simulink model "ADAS_Main_ClosedLoop"  (R2026a)
settings: Solver=FixedStepDiscrete  StopTime=20
InitFcn:
  | createLidarActorProfiles;
  | % L3/L4 closed-loop ego initial condition, READ FROM THE TEST-1 FIXTURE
  | % (not hard-coded in the vehicle model, which stays reusable)
  | clS = load('D:\AutonomousDriving\D_scenarios\V2_0_ClosedLoop_Test9_TwoObstacles_WideRoad.mat');
  | clA = clS.data.ActorSpecifications([clS.data.ActorSpecifications.ActorID] == clS.data.EgoCarId);
  | CL_EGO_IC = [clA.Position(1); clA.Position(2); clA.Yaw*pi/180; clA.Speed(1)];
  | clear clS clA
  | % Non-virtual ego-pose bus type. A MATLAB Function block (Extract_Ego_Kinematics)
  | % cannot accept a VIRTUAL bus, so the Bus Creator must emit a defined Simulink.Bus.
  | % Shape copied from the installed validator contract and from BusActorsActors.
  | clN = {'ActorID','Position','Velocity','Roll','Pitch','Yaw','AngularVelocity'};
  | clD = {[1 1],[1 3],[1 3],[1 1],[1 1],[1 1],[1 3]};
  | clEls = Simulink.BusElement.empty(0,1);
  | for clI = 1:7
  |   clE = Simulink.BusElement; clE.Name = clN{clI}; clE.Dimensions = clD{clI}; clE.DataType = 'double';
  |   clEls(clI,1) = clE;
  | end
  | BusEgoPose_CL = Simulink.Bus; BusEgoPose_CL.Elements = clEls;
  | clear clN clD clEls clE clI
StopFcn:
  | cl_plot_closedloop_trajectory;
model workspace (MAT data in the model file):
  firstWarning = 1
  originalScenarioChecksum = '71EAF3DF157DF5A35F75811B676F8B0F'
undefined symbols (not defined in the file): driving, matlabshared
libraries: drivingscenarioandsensors x3, lidarlib x1
(part 2 of 7)

== matlab function ADAS_Main_ClosedLoop/Sensor_Fusion/Normalize_Detections ==
  data: visionBus input; visionMeas output; radarBus input; lidarDet input; numLidarDet input; numVision output; radarMeas output; numRadar output; lidarMeas output; numLidar output
function [visionMeas, numVision, radarMeas, numRadar, lidarMeas, numLidar] = ...
    Normalize_Detections(visionBus, radarBus, lidarDet, numLidarDet)
%#codegen
% NORMALIZE_DETECTIONS  Stage F2 of Sensor Fusion: normalisation ONLY.
%
% Unpacks the Vision and Radar detection buses and the LiDAR detection matrix
% into three fixed-size measurement tables in the common ego frame.
%
% THIS STAGE DOES NOT: associate, gate, fuse, score, inflate covariance,
% classify, estimate velocity, or discard anything.
%
% NOTHING IS REJECTED. Every emitted detection is preserved. Covariance
% validity is reported per detection via CovValid flags so that the later
% fusion stage decides what to do. "no detection" and "detection with invalid
% covariance" are therefore never confused: the former has Valid = 0, the
% latter has Valid = 1 with PosCovValid = 0.
%
% MEASUREMENT SUBSPACES - only what each sensor actually measures:
%   Vision : x, y, vx, vy  (+ their 2x2 covariances)
%   Radar  : x, y, vx, vy  (+ their 2x2 covariances) + SNR
%   LiDAR  : the validated [256x20] detection row, passed through unchanged
%   Radar z / vz and Vision z / vz are NOT normalised. Radar elevation is off,
%   so its z is a nominal constant, not a measurement; vz is unobserved by both
%   (reported variance 100). Manufacturing them here would invent capability
%   the sensors do not have.
%
% SCENARIO INDEPENDENCE: reads only measurements and measurement covariance.
% It does not reference ActorID, ClassID, MaterialID, Clusters, actor poses,
% actor profiles, TargetIndex, or any scenario property. Loop bounds are the
% declared sensor interface capacities, never an actor count.

MAX_V  = 50;   NCOL_V = 13;   % Vision capacity  = MaxNumDetections
MAX_R  = 50;   NCOL_R = 14;   % Radar  capacity  = MaxNumReports
MAX_L  = 256;  NCOL_L = 21;   % LiDAR  capacity  = LiDARDetections rows

% Vision / Radar table columns
%   1 Valid
%   2 PosX          m
%   3 PosY          m
%   4 PosCovXX      m^2
%   5 PosCovYY      m^2
%   6 PosCovXY      m^2
%   7 VelX          m/s
%   8 VelY          m/s
%   9 VelCovXX      m^2/s^2
%  10 VelCovYY      m^2/s^2
%  11 VelCovXY      m^2/s^2
%  12 PosCovValid   0/1   2x2 position covariance is finite and positive definite
%  13 VelCovValid   0/1   2x2 velocity covariance is finite and positive definite
%  14 SNR           dB    (Radar table only)
%
% LiDAR table columns
%   1..20  the LiDARDetections row, unchanged
%   21     PosCovValid  0/1   from columns 5,6,7

visionMeas = zeros(MAX_V, NCOL_V);
radarMeas  = zeros(MAX_R, NCOL_R);
lidarMeas  = zeros(MAX_L, NCOL_L);

%% ---- Vision -------------------------------------------------------------
nV = double(visionBus.NumDetections);
if nV < 0,     nV = 0;     end
if nV > MAX_V, nV = MAX_V;  end
for i = 1:MAX_V
    if i > nV
        continue
    end
    m = visionBus.Detections(i).Measurement;
    C = visionBus.Detections(i).MeasurementNoise;
    pxx = double(C(1,1)); pyy = double(C(2,2)); pxy = double(C(1,2));
    vxx = double(C(4,4)); vyy = double(C(5,5)); vxy = double(C(4,5));
    visionMeas(i, 1)  = 1;
    visionMeas(i, 2)  = double(m(1));
    visionMeas(i, 3)  = double(m(2));
    visionMeas(i, 4)  = pxx;
    visionMeas(i, 5)  = pyy;
    visionMeas(i, 6)  = pxy;
    visionMeas(i, 7)  = double(m(4));
    visionMeas(i, 8)  = double(m(5));
    visionMeas(i, 9)  = vxx;
    visionMeas(i, 10) = vyy;
    visionMeas(i, 11) = vxy;
    if isPD2(pxx, pyy, pxy), visionMeas(i, 12) = 1; end
    if isPD2(vxx, vyy, vxy), visionMeas(i, 13) = 1; end
end
numVision = uint32(nV);

%% ---- Radar --------------------------------------------------------------
nR = double(radarBus.NumDetections);
if nR < 0,     nR = 0;     end
if nR > MAX_R, nR = MAX_R;  end
for i = 1:MAX_R
    if i > nR
        continue
    end
    m = radarBus.Detections(i).Measurement;
    C = radarBus.Detections(i).MeasurementNoise;
    pxx = double(C(1,1)); pyy = double(C(2,2)); pxy = double(C(1,2));
    vxx = double(C(4,4)); vyy = double(C(5,5)); vxy = double(C(4,5));
    radarMeas(i, 1)  = 1;
    radarMeas(i, 2)  = double(m(1));
    radarMeas(i, 3)  = double(m(2));
    radarMeas(i, 4)  = pxx;
    radarMeas(i, 5)  = pyy;
    radarMeas(i, 6)  = pxy;
    radarMeas(i, 7)  = double(m(4));
    radarMeas(i, 8)  = double(m(5));
    radarMeas(i, 9)  = vxx;
    radarMeas(i, 10) = vyy;
    radarMeas(i, 11) = vxy;
    if isPD2(pxx, pyy, pxy), radarMeas(i, 12) = 1; end
    if isPD2(vxx, vyy, vxy), radarMeas(i, 13) = 1; end
    % SNR only. No other ObjectAttributes field is read.
    radarMeas(i, 14) = double(radarBus.Detections(i).ObjectAttributes.SNR);
end
numRadar = uint32(nR);

%% ---- LiDAR --------------------------------------------------------------
nL = double(numLidarDet);
if nL < 0,     nL = 0;     end
if nL > MAX_L, nL = MAX_L;  end
for i = 1:MAX_L
    if i > nL
        continue
    end
    for c = 1:20
        lidarMeas(i, c) = lidarDet(i, c);
    end
    if isPD2(lidarDet(i,5), lidarDet(i,6), lidarDet(i,7))
        lidarMeas(i, 21) = 1;
    end
end
numLidar = uint32(nL);

end

% ===========================================================================
function tf = isPD2(a, b, c)
% 2x2 symmetric [a c; c b] is positive definite iff a > 0 and det > 0.
tf = false;
if isfinite(a) && isfinite(b) && isfinite(c)
    if a > 0 && b > 0 && (a*b - c*c) > 0
        tf = true;
    end
end
end

== matlab function ADAS_Main_ClosedLoop/Sensor_Fusion/Associate_Detections ==
  data: visionMeas input; groups output; numVision input; radarMeas input; numRadar input; lidarMeas input; numLidar input; numGroups output
function [groups, numGroups] = Associate_Detections( ...
    visionMeas, numVision, radarMeas, numRadar, lidarMeas, numLidar)
%#codegen
% ASSOCIATE_DETECTIONS  Stage F3: gating + compatibility grouping ONLY.
%
% THIS STAGE DOES NOT: fuse positions, fuse velocities, compute a support
% score, fuse class, or discard any detection. It only decides which sensor
% measurements are compatible enough to represent the same physical object.
%
% EVERY detection appears in exactly one group. A detection with no compatible
% partner forms a singleton group - that is the expected outcome for the large
% majority, because Radar and Vision have narrow forward fields of view while
% LiDAR is 360 deg. A high LiDAR count must never be forced into matches.
%
% GATE
%   2-D Mahalanobis on position only:
%       d2 = delta' * inv(R1' + R2') * delta        delta = [dx; dy]
%       compatible iff d2 < GATE_CHI2
%   Position only, because z is unobserved by Vision and nominal-only for
%   Radar, and velocity is unavailable from LiDAR.
%
% LiDAR REFERENCE-POINT TERM  B
%   LiDAR reports the centroid of visible surfaces, not the object centre.
%   Modelling that offset as uniform over the object's line-of-sight depth D
%   gives variance D^2/12 (the second moment of a uniform offset). Applied
%   ALONG the line of sight only, then rotated into ego coordinates.
%
%   Applied ONLY when ExtentUntrusted (LiDARFlags bit 8) is set. When the
%   extents are trustworthy the LiDAR block's own GAMMA_ALONG = 0.25 term is
%   already 87% of 1/(2*sqrt(3)) = 0.2887, i.e. it already implements
%   approximately this same variance using the yaw-projected depth
%   D_los = |L*cos(theta)| + |W*sin(theta)|, so adding B there would
%   double-count.
%
%   When ExtentUntrusted, the PCA extents have collapsed and that projection is
%   meaningless, so D_los = max(Length, Width) is used as a geometric proxy.
%   KNOWN LIMITATION: for a long object viewed end-on this under-estimates the
%   true line-of-sight depth.
%
% GROUPING
%   Mutual-best matching, which is symmetric and therefore order-independent:
%   a pair is joined only if each is the other's lowest-d2 compatible partner.
%   Ties break on the lower index. A group holds at most one detection per
%   sensor. Before a group keeps both a Vision and a Radar member they must
%   also be compatible with each other (clique, never a chain); if not, the
%   weaker link is dropped and ChainSplit is flagged.
%
% SCENARIO INDEPENDENCE: reads only measurements, covariances and LiDAR
% observation flags. No actor identity, class, count or scenario geometry.
% Loop bounds are the declared interface capacities.

MAX_V = 50; MAX_R = 50; MAX_L = 256; MAX_G = 356; NCOL_G = 6;
GATE_CHI2 = 9.21;        % chi-square, 2 DOF, 0.99

% LiDARMeas column map
CL_X = 2; CL_Y = 3; CL_CXX = 5; CL_CYY = 6; CL_CXY = 7;
CL_LEN = 9; CL_WID = 10; CL_FLAGS = 20; CL_COVOK = 21;
FLAG_EXTENT_UNTRUSTED = uint32(8);

groups    = zeros(MAX_G, NCOL_G);
numGroups = uint32(0);

nV = double(numVision); if nV > MAX_V, nV = MAX_V; end; if nV < 0, nV = 0; end
nR = double(numRadar);  if nR > MAX_R, nR = MAX_R; end; if nR < 0, nR = 0; end
nL = double(numLidar);  if nL > MAX_L, nL = MAX_L; end; if nL < 0, nL = 0; end

%% ---- gather positions, covariances and per-detection covariance validity
vx = zeros(MAX_V,1); vy = zeros(MAX_V,1);
vxx = zeros(MAX_V,1); vyy = zeros(MAX_V,1); vxy = zeros(MAX_V,1);
vok = false(MAX_V,1);
for i = 1:nV
    vx(i) = visionMeas(i,2);  vy(i) = visionMeas(i,3);
    vxx(i)= visionMeas(i,4);  vyy(i)= visionMeas(i,5);  vxy(i)= visionMeas(i,6);
    vok(i)= visionMeas(i,12) == 1;
end

rx = zeros(MAX_R,1); ry = zeros(MAX_R,1);
rxx = zeros(MAX_R,1); ryy = zeros(MAX_R,1); rxy = zeros(MAX_R,1);
rok = false(MAX_R,1);
for i = 1:nR
    rx(i) = radarMeas(i,2);  ry(i) = radarMeas(i,3);
    rxx(i)= radarMeas(i,4);  ryy(i)= radarMeas(i,5);  rxy(i)= radarMeas(i,6);
    rok(i)= radarMeas(i,12) == 1;
end

lx = zeros(MAX_L,1); ly = zeros(MAX_L,1);
lxx = zeros(MAX_L,1); lyy = zeros(MAX_L,1); lxy = zeros(MAX_L,1);
lok = false(MAX_L,1); lbias = false(MAX_L,1);
for i = 1:nL
    px = lidarMeas(i,CL_X);  py = lidarMeas(i,CL_Y);
    lx(i) = px;  ly(i) = py;
    cxx = lidarMeas(i,CL_CXX); cyy = lidarMeas(i,CL_CYY); cxy = lidarMeas(i,CL_CXY);
    if bitand(uint32(lidarMeas(i,CL_FLAGS)), FLAG_EXTENT_UNTRUSTED) > 0
        D = lidarMeas(i,CL_LEN);
        if lidarMeas(i,CL_WID) > D, D = lidarMeas(i,CL_WID); end
        bAlong = (D*D)/12;
        az = atan2(py, px);
        ca = cos(az); sa = sin(az);
        cxx = cxx + bAlong*ca*ca;
        cyy = cyy + bAlong*sa*sa;
        cxy = cxy + bAlong*ca*sa;
        lbias(i) = true;
    end
    lxx(i) = cxx; lyy(i) = cyy; lxy(i) = cxy;
    lok(i) = lidarMeas(i,CL_COVOK) == 1;
end

%% ---- pairwise gate
% A detection whose position covariance is not positive definite cannot be
% gated (the Mahalanobis distance is undefined), so it is never associated.
% It is preserved as a singleton and flagged, never discarded.
dVR = zeros(MAX_V, MAX_R); cVR = false(MAX_V, MAX_R);
dVL = zeros(MAX_V, MAX_L); cVL = false(MAX_V, MAX_L);
dRL = zeros(MAX_R, MAX_L); cRL = false(MAX_R, MAX_L);

for i = 1:nV
    for j = 1:nR
        if vok(i) && rok(j)
            [ok, d2] = gate2(vx(i)-rx(j), vy(i)-ry(j), ...
                vxx(i)+rxx(j), vyy(i)+ryy(j), vxy(i)+rxy(j), GATE_CHI2);
            dVR(i,j) = d2; cVR(i,j) = ok;
        end
    end
end
for i = 1:nV
    for j = 1:nL
        if vok(i) && lok(j)
            [ok, d2] = gate2(vx(i)-lx(j), vy(i)-ly(j), ...
                vxx(i)+lxx(j), vyy(i)+lyy(j), vxy(i)+lxy(j), GATE_CHI2);
            dVL(i,j) = d2; cVL(i,j) = ok;
        end
    end
end
for i = 1:nR
    for j = 1:nL
        if rok(i) && lok(j)
            [ok, d2] = gate2(rx(i)-lx(j), ry(i)-ly(j), ...
                rxx(i)+lxx(j), ryy(i)+lyy(j), rxy(i)+lxy(j), GATE_CHI2);
            dRL(i,j) = d2; cRL(i,j) = ok;
        end
    end
end

%% ---- mutual-best matching (symmetric => order-independent)
mVL = zeros(MAX_L,1);   % for each LiDAR, its mutually-best Vision (0 = none)
mRL = zeros(MAX_L,1);   % for each LiDAR, its mutually-best Radar
mVR = zeros(MAX_V,1);   % for each Vision, its mutually-best Radar

for j = 1:nL
    b = bestIn(dVL(:,j), cVL(:,j), nV);
    if b > 0
        bb = bestIn(dVL(b,:)', cVL(b,:)', nL);
        if bb == j, mVL(j) = b; end
    end
end
for j = 1:nL
    b = bestIn(dRL(:,j), cRL(:,j), nR);
    if b > 0
        bb = bestIn(dRL(b,:)', cRL(b,:)', nL);
        if bb == j, mRL(j) = b; end
    end
end
for i = 1:nV
    b = bestIn(dVR(i,:)', cVR(i,:)', nR);
    if b > 0
        bb = bestIn(dVR(:,b), cVR(:,b), nV);
        if bb == i, mVR(i) = b; end
    end
end

%% ---- build groups: LiDAR-anchored first, then leftover Radar/Vision
vUsed = false(MAX_V,1); rUsed = false(MAX_R,1);
g = 0;

for j = 1:nL
    g = g + 1;
    vIdx = mVL(j); rIdx = mRL(j);
    if vIdx > 0 && vUsed(vIdx), vIdx = 0; end
    if rIdx > 0 && rUsed(rIdx), rIdx = 0; end
    fl = 0;
    % clique: a group holding both Vision and Radar needs them compatible too
    if vIdx > 0 && rIdx > 0 && ~cVR(vIdx, rIdx)
        if dVL(vIdx,j) <= dRL(rIdx,j)
            rIdx = 0;
        else
            vIdx = 0;
        end
        fl = fl + 1;                       % ChainSplit
    end
    if ~lok(j), fl = fl + 2; end           % CovInvalid member
    if lbias(j), fl = fl + 4; end          % LiDAR B applied
    if vIdx > 0, vUsed(vIdx) = true; end
    if rIdx > 0, rUsed(rIdx) = true; end
    cnt = 1;
    if vIdx > 0, cnt = cnt + 1; end
    if rIdx > 0, cnt = cnt + 1; end
    groups(g,1) = 1;
    groups(g,2) = vIdx;
    groups(g,3) = rIdx;
    groups(g,4) = j;
    groups(g,5) = cnt;
    groups(g,6) = fl;
end

% Radar not yet grouped: may pair with an ungrouped mutually-best Vision
for i = 1:nR
    if rUsed(i), continue; end
    g = g + 1;
    vIdx = 0;
    for k = 1:nV
        if mVR(k) == i && ~vUsed(k)
            vIdx = k; break
        end
    end
    fl = 0;
    if ~rok(i), fl = fl + 2; end
    if vIdx > 0, vUsed(vIdx) = true; end
    cnt = 1; if vIdx > 0, cnt = 2; end
    groups(g,1) = 1;
    groups(g,2) = vIdx;
    groups(g,3) = i;
    groups(g,4) = 0;
    groups(g,5) = cnt;
    groups(g,6) = fl;
    rUsed(i) = true;
end

% Vision left over: singletons
for i = 1:nV
    if vUsed(i), continue; end
    g = g + 1;
    fl = 0;
    if ~vok(i), fl = fl + 2; end
    groups(g,1) = 1;
    groups(g,2) = i;
    groups(g,3) = 0;
    groups(g,4) = 0;
    groups(g,5) = 1;
    groups(g,6) = fl;
    vUsed(i) = true;
end

numGroups = uint32(g);

end

% ===========================================================================
function [ok, d2] = gate2(dx, dy, sxx, syy, sxy, thr)
ok = false; d2 = 0;
det = sxx*syy - sxy*sxy;
if isfinite(det) && det > 0 && sxx > 0
    d2 = (dx*dx*syy - 2*dx*dy*sxy + dy*dy*sxx)/det;
    if isfinite(d2) && d2 >= 0 && d2 < thr
        ok = true;
    end
end
end

% ===========================================================================
function b = bestIn(d, c, n)
% Lowest d2 among compatible entries 1..n. Ties break on the lower index.
b = 0; bd = 0;
for k = 1:n
    if c(k)
        if b == 0 || d(k) < bd
            b = k; bd = d(k);
        end
    end
end
end

== matlab function ADAS_Main_ClosedLoop/Sensor_Fusion/Fuse_Position ==
  data: visionMeas input; fusedPos output; numVision input; radarMeas input; numRadar input; lidarMeas input; numLidar input; groups input; numGroups input; numFused output
function [fusedPos, numFused] = Fuse_Position( ...
    visionMeas, numVision, radarMeas, numRadar, lidarMeas, numLidar, groups, numGroups)
%#codegen
% FUSE_POSITION  Stage F4: information-form fusion of X/Y position ONLY.
%
% THIS STAGE DOES NOT: fuse velocity, compute a support score, fuse class,
% track, or discard anything. Every group from F3 produces exactly one output
% row, in the same order.
%
% METHOD
%   For a group with two or more usable members, the maximum-likelihood
%   combination of independent simultaneous measurements is the information
%   form:
%       Y = sum_i inv(Ri)          (information matrix)
%       y = sum_i inv(Ri) * zi     (information vector)
%       P = inv(Y),  x = P * y
%   For a singleton the measurement and covariance pass through unchanged.
%   There is no prediction, no process model and no state carried between
%   frames - that belongs to Tracking, not here.
%
% LiDAR REFERENCE-POINT TERM  B
%   Recomputed here with the SAME formula used by Associate_Detections in F3:
%   applied only when ExtentUntrusted (LiDARFlags bit 8), D = max(Length,Width),
%   variance D^2/12 along the line of sight, rotated into ego coordinates.
%   The two stages must stay in sync; the F4 checkpoint verifies this by
%   recomputing B independently and comparing the singleton LiDAR rows.
%
% DEFENSIVE COVARIANCE HANDLING
%   A member whose 2x2 position covariance is not finite and positive definite
%   is NEVER inverted. It is excluded from the information sum and
%   FusionDegraded is flagged. If no member has a usable covariance the
%   detection is still preserved: its raw position is passed through with its
%   own covariance untouched, and the flags say so. Nothing is discarded and
%   no singular matrix is ever used.
%
% SCENARIO INDEPENDENCE: consumes only measurements, covariances, LiDAR
% observation flags and the F3 grouping. No actor identity, class, count or
% scenario geometry. Loop bounds are the declared interface capacities.

MAX_G = 356; NCOL_F = 11;
FLAG_EXTENT_UNTRUSTED = uint32(8);

% LiDARMeas column map
CL_X = 2; CL_Y = 3; CL_CXX = 5; CL_CYY = 6; CL_CXY = 7;
CL_LEN = 9; CL_WID = 10; CL_FLAGS = 20;

% fusedPos columns
%   1 Valid
%   2 PosX          m, ego
%   3 PosY          m, ego
%   4 PosCovXX      m^2
%   5 PosCovYY      m^2
%   6 PosCovXY      m^2
%   7 SensorMask    1 = Vision, 2 = Radar, 4 = LiDAR
%   8 VisionIdx     source row in visionMeas (0 = none)
%   9 RadarIdx      source row in radarMeas  (0 = none)
%  10 LiDARIdx      source row in lidarMeas  (0 = none)
%  11 FusionFlags   1 ChainSplit | 2 CovInvalidMember | 4 LiDARBiasApplied
%                   8 FusionDegraded | 16 OutsideMeasurementBox

fusedPos = zeros(MAX_G, NCOL_F);
numFused = uint32(0);

nG = double(numGroups);
if nG < 0, nG = 0; end
if nG > MAX_G, nG = MAX_G; end

for g = 1:nG
    if groups(g,1) ~= 1
        continue
    end
    vi = groups(g,2);
    ri = groups(g,3);
    li = groups(g,4);
    fl = uint32(groups(g,6));        % inherit ChainSplit / CovInvalid / BiasApplied

    % ---- gather up to three members
    mx = zeros(3,1); my = zeros(3,1);
    ma = zeros(3,1); mb = zeros(3,1); mc = zeros(3,1);
    mUse = false(3,1);
    nMem = 0;
    mask = 0;

    if vi > 0
        nMem = nMem + 1; mask = mask + 1;
        mx(nMem) = visionMeas(vi,2); my(nMem) = visionMeas(vi,3);
        ma(nMem) = visionMeas(vi,4); mb(nMem) = visionMeas(vi,5); mc(nMem) = visionMeas(vi,6);
        mUse(nMem) = isPD2(ma(nMem), mb(nMem), mc(nMem));
    end
    if ri > 0
        nMem = nMem + 1; mask = mask + 2;
        mx(nMem) = radarMeas(ri,2); my(nMem) = radarMeas(ri,3);
        ma(nMem) = radarMeas(ri,4); mb(nMem) = radarMeas(ri,5); mc(nMem) = radarMeas(ri,6);
        mUse(nMem) = isPD2(ma(nMem), mb(nMem), mc(nMem));
    end
    if li > 0
        nMem = nMem + 1; mask = mask + 4;
        px = lidarMeas(li,CL_X); py = lidarMeas(li,CL_Y);
        a = lidarMeas(li,CL_CXX); b = lidarMeas(li,CL_CYY); c = lidarMeas(li,CL_CXY);
        if bitand(uint32(lidarMeas(li,CL_FLAGS)), FLAG_EXTENT_UNTRUSTED) > 0
            D = lidarMeas(li,CL_LEN);
            if lidarMeas(li,CL_WID) > D, D = lidarMeas(li,CL_WID); end
            bAlong = (D*D)/12;
            az = atan2(py, px);
            ca = cos(az); sa = sin(az);
            a = a + bAlong*ca*ca;
            b = b + bAlong*sa*sa;
            c = c + bAlong*ca*sa;
        end
        mx(nMem) = px; my(nMem) = py;
        ma(nMem) = a;  mb(nMem) = b;  mc(nMem) = c;
        mUse(nMem) = isPD2(a, b, c);
    end

    nUse = 0;
    for m = 1:nMem
        if mUse(m), nUse = nUse + 1; end
    end
    if nUse < nMem
        fl = fl + uint32(8);                     % FusionDegraded
    end

    outX = 0; outY = 0; outA = 0; outB = 0; outC = 0;

    if nUse == 0
        % preserve the detection; never invert a singular matrix
        outX = mx(1); outY = my(1);
        outA = ma(1); outB = mb(1); outC = mc(1);
    elseif nUse == 1
        for m = 1:nMem
            if mUse(m)
                outX = mx(m); outY = my(m);
                outA = ma(m); outB = mb(m); outC = mc(m);
            end
        end
    else
        % ---- information form over the usable members
        Yxx = 0; Yyy = 0; Yxy = 0; yx = 0; yy = 0;
        for m = 1:nMem
            if ~mUse(m), continue; end
            det = ma(m)*mb(m) - mc(m)*mc(m);
            ixx =  mb(m)/det;
            iyy =  ma(m)/det;
            ixy = -mc(m)/det;
            Yxx = Yxx + ixx;
            Yyy = Yyy + iyy;
            Yxy = Yxy + ixy;
            yx = yx + ixx*mx(m) + ixy*my(m);
            yy = yy + ixy*mx(m) + iyy*my(m);
        end
        dY = Yxx*Yyy - Yxy*Yxy;
        if isfinite(dY) && dY > 0 && Yxx > 0
            outA =  Yyy/dY;
            outB =  Yxx/dY;
            outC = -Yxy/dY;
            outX = outA*yx + outC*yy;
            outY = outC*yx + outB*yy;
        else
            % should be unreachable: a sum of PD matrices is PD
            fl = fl + uint32(8);
            for m = 1:nMem
                if mUse(m)
                    outX = mx(m); outY = my(m);
                    outA = ma(m); outB = mb(m); outC = mc(m);
                    break
                end
            end
        end

        % ---- bounding-box check over the contributing measurements
        loX = mx(1); hiX = mx(1); loY = my(1); hiY = my(1);
        first = true;
        for m = 1:nMem
            if ~mUse(m), continue; end
            if first
                loX = mx(m); hiX = mx(m); loY = my(m); hiY = my(m); first = false;
            else
                if mx(m) < loX, loX = mx(m); end
                if mx(m) > hiX, hiX = mx(m); end
                if my(m) < loY, loY = my(m); end
                if my(m) > hiY, hiY = my(m); end
            end
        end
        tol = 1e-9;
        if outX < loX-tol || outX > hiX+tol || outY < loY-tol || outY > hiY+tol
            fl = fl + uint32(16);                % OutsideMeasurementBox
        end
    end

    fusedPos(g, 1)  = 1;
    fusedPos(g, 2)  = outX;
    fusedPos(g, 3)  = outY;
    fusedPos(g, 4)  = outA;
    fusedPos(g, 5)  = outB;
    fusedPos(g, 6)  = outC;
    fusedPos(g, 7)  = mask;
    fusedPos(g, 8)  = vi;
    fusedPos(g, 9)  = ri;
    fusedPos(g, 10) = li;
    fusedPos(g, 11) = double(fl);
end

numFused = uint32(nG);

end

% ===========================================================================
function tf = isPD2(a, b, c)
tf = false;
if isfinite(a) && isfinite(b) && isfinite(c)
    if a > 0 && b > 0 && (a*b - c*c) > 0
        tf = true;
    end
end
end

== matlab function ADAS_Main_ClosedLoop/Sensor_Fusion/Fuse_Velocity ==
  data: visionMeas input; fusedVel output; numVision input; radarMeas input; numRadar input; fusedPos input; numFused input; numFusedVel output
function [fusedVel, numFusedVel] = Fuse_Velocity( ...
    visionMeas, numVision, radarMeas, numRadar, fusedPos, numFused)
%#codegen
% FUSE_VELOCITY  Stage F5: velocity SELECTION (not fusion).
%
% Velocity is deliberately NOT combined across sensors, unlike position.
% Two measured facts rule out an information-form combination:
%   1. The Vision generator's velocity covariance DIVERGES with time
%      (1.04 -> 3.53 m^2/s^2 over 2.4 s and still rising). It is an internal
%      estimator covariance, not a stationary measurement noise, so it is not
%      a valid R.
%   2. Both generators emit internally FILTERED velocity, so the two are not
%      independent measurements at a timestep. Information-form fusion assumes
%      independence and would be invalid.
%
% Policy: Radar primary, Vision as fallback only, never blended.
%   - If the Radar member has a usable velocity covariance, its velocity and
%     covariance are copied EXACTLY. If Vision is also present, a consistency
%     gate is evaluated and flagged - but the estimate stays Radar's.
%   - Otherwise, if the Vision member has a usable velocity covariance, its
%     velocity and covariance are copied EXACTLY.
%   - Otherwise the object carries no velocity measurement.
%
% UNOBSERVED CONVENTION
%   VelX = VelY = 0 and VelCovXX = VelCovYY = VelCovXY = 0 with bit 4
%   (VelUnobserved) set means "NO VELOCITY MEASUREMENT" - it does NOT mean a
%   stationary object known with perfect certainty. This matches the convention
%   already used for HeightAboveGround = 0 with GroundUnavailable, and for
%   ObjectClassID = 0 meaning "not populated". Downstream MUST test bit 4
%   before using velocity. LiDAR supplies no velocity, so LiDAR-only objects
%   always carry bit 4; estimating their velocity belongs to Tracking.
%
% A covariance that is not finite and positive definite is NEVER inverted and
% is never emitted as if usable.
%
% SCENARIO INDEPENDENCE: consumes only measurements, covariances and the F4
% provenance. No actor identity, class, count or scenario geometry.

MAX_G = 356; NCOL_V = 7;
GATE_CHI2 = 9.21;          % chi-square, 2 DOF, 0.99

% visionMeas / radarMeas velocity columns
CV_VX = 7; CV_VY = 8; CV_XX = 9; CV_YY = 10; CV_XY = 11; CV_OK = 13;
% fusedPos provenance columns
CF_VI = 8; CF_RI = 9;

% fusedVel columns
%   1 Valid
%   2 VelX       m/s, ego
%   3 VelY       m/s, ego
%   4 VelCovXX   m^2/s^2
%   5 VelCovYY   m^2/s^2
%   6 VelCovXY   m^2/s^2
%   7 VelFlags   1 VelFromRadar | 2 VelFromVisionOnly | 4 VelUnobserved
%                8 VelCovInvalidRejected | 16 VelConsistencyFail

fusedVel = zeros(MAX_G, NCOL_V);
numFusedVel = uint32(0);

nG = double(numFused);
if nG < 0, nG = 0; end
if nG > MAX_G, nG = MAX_G; end

for g = 1:nG
    if fusedPos(g,1) ~= 1
        continue
    end
    vi = fusedPos(g, CF_VI);
    ri = fusedPos(g, CF_RI);

    radarOK  = false;
    visionOK = false;
    if ri > 0
        radarOK = isPD2(radarMeas(ri,CV_XX), radarMeas(ri,CV_YY), radarMeas(ri,CV_XY));
    end
    if vi > 0
        visionOK = isPD2(visionMeas(vi,CV_XX), visionMeas(vi,CV_YY), visionMeas(vi,CV_XY));
    end

    vx = 0; vy = 0; cxx = 0; cyy = 0; cxy = 0;
    fl = uint32(0);

    if radarOK
        % exact copy - no blending, no inflation
        vx  = radarMeas(ri,CV_VX);
        vy  = radarMeas(ri,CV_VY);
        cxx = radarMeas(ri,CV_XX);
        cyy = radarMeas(ri,CV_YY);
        cxy = radarMeas(ri,CV_XY);
        fl  = fl + uint32(1);                       % VelFromRadar

        if visionOK
            % consistency gate only; the estimate remains Radar's
            dvx = radarMeas(ri,CV_VX) - visionMeas(vi,CV_VX);
            dvy = radarMeas(ri,CV_VY) - visionMeas(vi,CV_VY);
            sxx = radarMeas(ri,CV_XX) + visionMeas(vi,CV_XX);
            syy = radarMeas(ri,CV_YY) + visionMeas(vi,CV_YY);
            sxy = radarMeas(ri,CV_XY) + visionMeas(vi,CV_XY);
            det = sxx*syy - sxy*sxy;
            if isfinite(det) && det > 0 && sxx > 0
                d2 = (dvx*dvx*syy - 2*dvx*dvy*sxy + dvy*dvy*sxx)/det;
                if ~(isfinite(d2) && d2 < GATE_CHI2)
                    fl = fl + uint32(16);           % VelConsistencyFail
                end
            else
                fl = fl + uint32(16);
            end
        elseif vi > 0
            fl = fl + uint32(8);                    % a Vision velocity existed but was unusable
        end

    elseif visionOK
        vx  = visionMeas(vi,CV_VX);
        vy  = visionMeas(vi,CV_VY);
        cxx = visionMeas(vi,CV_XX);
        cyy = visionMeas(vi,CV_YY);
        cxy = visionMeas(vi,CV_XY);
        fl  = fl + uint32(2);                       % VelFromVisionOnly
        if ri > 0
            fl = fl + uint32(8);                    % Radar velocity existed but was unusable
        end

    else
        % no usable velocity source: zeros, flagged
        fl = fl + uint32(4);                        % VelUnobserved
        if vi > 0 || ri > 0
            fl = fl + uint32(8);                    % a source existed but its covariance was not PD
        end
    end

    fusedVel(g,1) = 1;
    fusedVel(g,2) = vx;
    fusedVel(g,3) = vy;
    fusedVel(g,4) = cxx;
    fusedVel(g,5) = cyy;
    fusedVel(g,6) = cxy;
    fusedVel(g,7) = double(fl);
end

numFusedVel = uint32(nG);

end

% ===========================================================================
function tf = isPD2(a, b, c)
tf = false;
if isfinite(a) && isfinite(b) && isfinite(c)
    if a > 0 && b > 0 && (a*b - c*c) > 0
        tf = true;
    end
end
end

== matlab function ADAS_Main_ClosedLoop/Sensor_Fusion/Assemble_FusedObjects ==
  data: fusedPos input; fusedObjects output; numFused input; fusedVel input; lidarMeas input; radarMeas input; numFusedObjects output
function [fusedObjects, numFusedObjects] = Assemble_FusedObjects( ...
    fusedPos, numFused, fusedVel, lidarMeas, radarMeas)
%#codegen
% ASSEMBLE_FUSEDOBJECTS  Stage F7: final assembly of the Sensor Fusion output.
%
% THIS STAGE DOES NOT: associate, fuse, filter, track, classify, reject or
% reorder anything. Every row produced by F4 becomes exactly one output row, in
% the same order and with the same index. The only value COMPUTED here is
% DetectionSupportScore (column 23); everything else is a copy of an already
% validated upstream value or a documented zero.
%
% PROVENANCE
%   Group g's contributing detections are named by the F4 provenance columns:
%       vi = fusedPos(g,8)   row in visionMeas   (0 = none)
%       ri = fusedPos(g,9)   row in radarMeas    (0 = none)
%       li = fusedPos(g,10)  row in lidarMeas    (0 = none)
%   These are copied verbatim from Groups(g,2:4) by F4, and lidarMeas(:,1:20)
%   is bit-identical to LiDARDetections, so lidarMeas(li,:) IS the contributing
%   LiDAR detection. No lookup, search or matching is performed here.
%
% NO-LiDAR-MEMBER CONVENTION
%   Columns 4, 8, 14..21 and 26 are LiDAR-derived. When li == 0 they are ALL
%   set to exactly 0. Zero in those columns therefore means "no LiDAR member",
%   NOT a measured zero. The unambiguous discriminator is column 8:
%   Extract_Object_Features floors PosCovZZ at 0.05^2 = 0.0025, so a real LiDAR
%   detection can never report 0 there. SensorMask bit 4 (column 22) must agree.
%   Column 26 alone is NOT a valid discriminator: LiDARFlags == 0 is a
%   legitimate value for a clean LiDAR detection.
%   NO LiDAR INFORMATION IS EVER MANUFACTURED FOR RADAR/VISION-ONLY OBJECTS.
%
% UNPOPULATED-CLASS CONVENTION
%   Columns 24 (ObjectClassID) and 25 (ClassConfidence) are hard zero, meaning
%   "not populated by the current Sensor Fusion implementation". Column 24 is
%   NOT class 0 and column 25 is NOT a confidence of zero. Classification has
%   no source in this pipeline: LiDAR geometry cannot supply it and the Vision
%   generator's ObjectClassParameters is empty.
%
% DETECTION SUPPORT SCORE (column 23)
%   S = 1 - (1-s_L)*(1-s_R), a noisy-OR over the only two per-detection quality
%   metrics that exist in this pipeline. Vision contributes NOTHING: it exposes
%   no per-detection quality, so there is no honest s_V to compute.
%     s_L = LiDAR Confidence (geometric detectability, already in [0,1])
%     s_R = (SNR_dB - SNR_FLOOR)/SNR_SPAN, clamped to [0,1]
%   SNR_FLOOR = 13.11 dB is SENSOR-DERIVED: Albersheim's equation applied to
%   the radar block's own DetectionProbability 0.9 and FalseAlarmRate 1e-6.
%   SNR_SPAN = 10 dB is an ENGINEERING DESIGN CHOICE: detection probability
%   rises from threshold to near unity within roughly 10 dB. Neither constant
%   is tuned to any scenario's observed SNR distribution.
%
%   S IS A QUALITY SIGNAL ONLY. Specifically:
%     - SNR below SNR_FLOOR drives s_R to 0 FOR THE SUPPORT SCORE ONLY.
%     - It does NOT reject the Radar detection; it stays Valid.
%     - It does NOT reduce the Radar member's contribution to position or
%       velocity fusion. F4 weights by inv(R) and F5 copies Radar exactly;
%       neither block reads SNR at all.
%     - S == 0 does NOT mean the detection is false, invalid or absent. It
%       means no contributing sensor exposed a usable per-detection quality
%       metric. Vision-only objects legitimately always score 0.
%     - Valid (column 1) and SensorMask (column 22) are the AUTHORITATIVE
%       presence indicators. Downstream MUST NOT gate on S alone.
%
% FUSIONFLAGS (column 27) - 10-bit lossless merge
%   Two upstream 5-bit fields are carried in one column. Bits 1..16 keep their
%   F4 meaning, value and name exactly; the F5 velocity bits are shifted left
%   by 5. Nothing is dropped, renumbered or repurposed.
%       1 ChainSplit            32 VelFromRadar
%       2 CovInvalidMember      64 VelFromVisionOnly
%       4 LiDARBiasApplied     128 VelUnobserved
%       8 FusionDegraded       256 VelCovInvalidRejected
%      16 OutsideMeasurementBox 512 VelConsistencyFail
%   Built with bitand/bitshift/bitor, never arithmetic addition, so the field
%   is bounded at 1023 by construction and cannot be corrupted by a double-add
%   upstream.
%   CONTRACT: test individual bits with bitand. NEVER test FusionFlags == 0.
%   Exactly one of bits 32/64/128 always fires, so column 27 is never zero.
%   Bit 128 (VelUnobserved) means columns 9..13 are zeros, NOT a measured
%   standstill. Tracking MUST test it before using velocity.
%
% SCENARIO INDEPENDENCE: consumes only upstream fused values, LiDAR geometry
% and Radar SNR. No actor identity, class, count, trajectory or scenario
% geometry. Loop bounds are the declared interface capacities.

MAX_G = 356; NCOL_O = 27;
MAX_L = 256; MAX_R = 50;

SNR_FLOOR = 13.11;        % dB, Albersheim from P_D = 0.9, P_FA = 1e-6
SNR_SPAN  = 10.0;         % dB, engineering design choice

% lidarMeas column map (cols 1..20 are bit-identical to LiDARDetections)
CL_Z = 4; CL_CZZ = 8; CL_LEN = 9; CL_WID = 10; CL_HGT = 11; CL_YAW = 12;
CL_ZB = 13; CL_HAG = 14; CL_CX = 15; CL_CY = 16; CL_CONF = 19; CL_FLAGS = 20;
% radarMeas column map
CR_SNR = 14;
% fusedPos column map
CP_VALID = 1; CP_X = 2; CP_Y = 3; CP_CXX = 4; CP_CYY = 5; CP_CXY = 6;
CP_MASK = 7; CP_RI = 9; CP_LI = 10; CP_FLAGS = 11;
% fusedVel column map
CV_VALID = 1; CV_VX = 2; CV_VY = 3; CV_CXX = 4; CV_CYY = 5; CV_CXY = 6;
CV_FLAGS = 7;

FLAG_MASK5     = uint32(31);
VEL_UNOBSERVED = uint32(4);      % F5 bit 4, before the shift

fusedObjects    = zeros(MAX_G, NCOL_O);
numFusedObjects = uint32(0);

nG = double(numFused);
if nG < 0, nG = 0; end
if nG > MAX_G, nG = MAX_G; end

for g = 1:nG
    if fusedPos(g, CP_VALID) ~= 1
        continue
    end

    ri = fusedPos(g, CP_RI);
    li = fusedPos(g, CP_LI);

    % ---- bound the provenance indices before any indexing (codegen safety)
    liOK = false;
    if li >= 1 && li <= MAX_L
        liOK = true;
    end
    riOK = false;
    if ri >= 1 && ri <= MAX_R
        riOK = true;
    end

    % ---- position: straight copy from F4
    fusedObjects(g, 1) = 1;
    fusedObjects(g, 2) = fusedPos(g, CP_X);
    fusedObjects(g, 3) = fusedPos(g, CP_Y);
    fusedObjects(g, 5) = fusedPos(g, CP_CXX);
    fusedObjects(g, 6) = fusedPos(g, CP_CYY);
    fusedObjects(g, 7) = fusedPos(g, CP_CXY);

    % ---- velocity: straight copy from F5, same row index
    velFl = uint32(0);
    if fusedVel(g, CV_VALID) == 1
        fusedObjects(g,  9) = fusedVel(g, CV_VX);
        fusedObjects(g, 10) = fusedVel(g, CV_VY);
        fusedObjects(g, 11) = fusedVel(g, CV_CXX);
        fusedObjects(g, 12) = fusedVel(g, CV_CYY);
        fusedObjects(g, 13) = fusedVel(g, CV_CXY);
        velFl = bitand(uint32(fusedVel(g, CV_FLAGS)), FLAG_MASK5);
    else
        % unreachable by construction: F5 emits one valid row per F4 row.
        % If it ever happened, zeros with VelUnobserved is the honest report.
        velFl = VEL_UNOBSERVED;
    end

    % ---- LiDAR-derived columns, or the documented all-zero convention
    sL = 0;
    if liOK
        fusedObjects(g,  4) = lidarMeas(li, CL_Z);
        fusedObjects(g,  8) = lidarMeas(li, CL_CZZ);
        fusedObjects(g, 14) = lidarMeas(li, CL_LEN);
        fusedObjects(g, 15) = lidarMeas(li, CL_WID);
        fusedObjects(g, 16) = lidarMeas(li, CL_HGT);
        fusedObjects(g, 17) = lidarMeas(li, CL_YAW);
        fusedObjects(g, 18) = lidarMeas(li, CL_ZB);
        fusedObjects(g, 19) = lidarMeas(li, CL_HAG);
        fusedObjects(g, 20) = lidarMeas(li, CL_CX);
        fusedObjects(g, 21) = lidarMeas(li, CL_CY);
        fusedObjects(g, 26) = lidarMeas(li, CL_FLAGS);
        sL = lidarMeas(li, CL_CONF);
        if ~isfinite(sL) || sL < 0, sL = 0; end
        if sL > 1, sL = 1; end
    end
    % else: columns 4, 8, 14..21, 26 stay exactly 0 - "no LiDAR member"

    % ---- provenance
    fusedObjects(g, 22) = fusedPos(g, CP_MASK);

    % ---- DetectionSupportScore
    sR = 0;
    if riOK
        snr = radarMeas(ri, CR_SNR);
        if isfinite(snr)
            sR = (snr - SNR_FLOOR) / SNR_SPAN;
            if sR < 0, sR = 0; end
            if sR > 1, sR = 1; end
        end
    end
    fusedObjects(g, 23) = 1 - (1 - sL) * (1 - sR);

    % ---- columns 24/25 remain exactly 0: "not populated", not class 0

    % ---- FusionFlags: lossless 10-bit merge, bitwise only
    posFl = bitand(uint32(fusedPos(g, CP_FLAGS)), FLAG_MASK5);
    fusedObjects(g, 27) = double(bitor(posFl, bitshift(velFl, 5)));
end

numFusedObjects = uint32(nG);

end

== matlab function ADAS_Main_ClosedLoop/Ego_Kinematics/Extract_Ego_Kinematics ==
  data: egoActor input; egoKin output
function egoKin = Extract_Ego_Kinematics(egoActor)
%#codegen
% EXTRACT_EGO_KINEMATICS  Ego bus -> the two kinematic scalars Tracking may use.
%
% PURPOSE
%   Structurally enforce the "no global ego pose" rule. This block is the ONLY
%   consumer of the ego bus. It reads exactly two fields and emits two scalars,
%   so Tracking_Prediction never receives Position, Yaw, Orientation or any
%   other global quantity - it cannot use them because it never sees them.
%
% READS  (and nothing else)
%   egoActor.Velocity(1:2)     m/s,   ground speed components
%   egoActor.AngularVelocity(3) deg/s, yaw rate about the vertical axis
%
% DELIBERATELY NOT READ
%   Position, Yaw, Roll, Pitch, ActorID, Velocity(3), AngularVelocity(1:2)
%
% UNITS - VERIFIED, NOT ASSUMED
%   Measured against a scenario with an exactly known yaw rate (circular path,
%   R = 50 m, v = 15 m/s => omega = v/R = 0.300000 rad/s = 17.1887 deg/s):
%       engine reported AngularVelocity(3) = 17.188734
%       reported / (deg/s expectation) = 1.0000
%       reported / (rad/s expectation)  = 57.2958  ( = 180/pi )
%   => AngularVelocity is in DEG/s. Yaw likewise in degrees (cross-checked).
%   => Velocity is in m/s (reported |v| = 15.000000 against 15 expected).
%
%   The deg -> rad conversion is applied HERE, EXACTLY ONCE. No downstream
%   block may convert again.
%
% OUTPUT
%   egoKin(1) = speed   m/s     = norm(Velocity(1:2))   - frame-invariant magnitude
%   egoKin(2) = yawRate rad/s   = AngularVelocity(3)*pi/180
%
% SCENARIO INDEPENDENCE: consumes only ego self-kinematics, the same class as
% wheel odometry + IMU on real hardware. No actor identity, class, count,
% trajectory, map or scenario geometry.

DEG2RAD = pi/180;

egoKin = zeros(1,2);

vx = egoActor.Velocity(1);
vy = egoActor.Velocity(2);
if ~isfinite(vx), vx = 0; end
if ~isfinite(vy), vy = 0; end
egoKin(1) = sqrt(vx*vx + vy*vy);

wz = egoActor.AngularVelocity(3);
if ~isfinite(wz), wz = 0; end
egoKin(2) = wz * DEG2RAD;

end

== matlab function ADAS_Main_ClosedLoop/Tracking_Prediction/Tracking_State_Update ==
  data: fusedObjects input; trkState output; numFusedObjects input; egoKin input; prevState input double size=512 4; prevCov input double size=512 10; prevID input uint32 size=512 1; prevStatus input uint8 size=512 1; prevNextID input uint32 size=1 1; trkCov output; trkID output; trkStatus output; nextID output; egoTransform output; predDiag output
function [trkState, trkCov, trkID, trkStatus, nextID, egoTransform, predDiag] = ...
    Tracking_State_Update(fusedObjects, numFusedObjects, egoKin, ...
                          prevState, prevCov, prevID, prevStatus, prevNextID)
%#codegen
% TRACKING_STATE_UPDATE  Stage 1 + Stage 2.
%   Stage 1: fixed-size track-state memory + exact ego-motion compensation.
%   Stage 2: constant-velocity prediction with DWNA process noise.
%
% THIS BLOCK STILL DOES NOT: associate, gate, match, create tracks, update from
% measurements, run a lifecycle, keep history, or emit prediction horizons.
% fusedObjects / numFusedObjects remain wired but UNCONSUMED; they are the
% frozen interface for Stage 3.
%
% ORDER OF OPERATIONS  (frozen architecture: compensate, then predict)
%   1. ego-motion compensation       x <- T*(x - d)      P <- T*P*T'
%   2. ego-motion uncertainty        P <- P + ego terms
%   3. constant-velocity prediction  x <- F*x            P <- F*P*F' + Q
%   4. symmetrise, floor, PD check, reset if required
%   VERIFIED: steps 1 and 3 commute exactly. F and T commute (T*F - F*T = 0)
%   and the isotropic Q is rotation invariant (max|T*Q*T' - Q| = 6.8e-21), so
%   the stated ordering is mathematically identical to the reverse. Measured
%   over 2000 random cases: max state diff 2.8e-14, max covariance diff 7.1e-15.
%
% STATE LAYOUT  (fixed-size, explicit Unit Delay feedback; no persistent vars)
%   trkState  [512 x 4]  double  X, Y, Vx, Vy            (ego frame)
%   trkCov    [512 x 10] double  upper triangle of symmetric 4x4 P, packed
%                                [P11 P12 P13 P14 P22 P23 P24 P33 P34 P44]
%   trkID     [512 x 1]  uint32  future persistent TrackID; 0 = unassigned
%   trkStatus [512 x 1]  uint8   0 = FREE SLOT. Stage 2 still only ever holds 0.
%   nextID    [1 x 1]    uint32  monotonic allocator, starts at 1, never reused
%   predDiag  [1 x 3]    double  [nActive, nCovFloored, nCovReset]
%
% SLOT INDEX IS NOT TRACK IDENTITY. Persistent identity is trkID, allocated from
% nextID once association exists (Stage 3+). NO TRACK CREATION OR IDENTITY
% ASSOCIATION IS IMPLEMENTED HERE.
%
% ZEROS ARE NOT MEASUREMENTS. A slot is meaningless unless trkStatus > 0. The
% all-zero state is UNOCCUPIED MEMORY, not a measured position and not a
% measured zero velocity.
%
% EGO-MOTION COMPENSATION - exact constant-turn-rate arc
%   |w| >  YAW_EPS :  dx = (v/w)*sin(w*dt) ,  dy = (v/w)*(1-cos(w*dt))
%   |w| <= YAW_EPS :  dx = v*dt            ,  dy = 0
%   dpsi = w*dt ; p_new = R(-dpsi)*(p_old-[dx;dy]) ; v_new = R(-dpsi)*v_old
%   Pure rigid re-expression. Translation does not act on velocity.
%   NO SIDESLIP MODEL: egoKin(1) is ground-speed magnitude acting along body x.
%
% PROCESS NOISE - DWNA, exactly the frozen form; q = SIGMA_A^2, units m^2/s^4.
%   qx = qy = 9.0 m^2/s^4 (SIGMA_A = 3.0 m/s^2).
%   Isotropic BY DESIGN: x and y are EGO-FRAME axes, not the tracked object's
%   longitudinal/lateral axes. Anisotropic q would assert every object is
%   aligned with the ego heading - false for crossing pedestrians, bicycles and
%   oncoming traffic - and would require a heading we cannot reliably observe.
%
% COVARIANCE DISCIPLINE
%   symmetrise every step; floor the diagonal; test positive definiteness of the
%   2x2 position and velocity blocks with the validated analytic check - never
%   inv(), never Inf/NaN sentinels. On failure, fall back to the floored
%   diagonal (guaranteed PD) and count it in predDiag(3).
%
% SCENARIO INDEPENDENCE: consumes only ego self-kinematics and its own prior
% state. No actor identity, class, count, trajectory, map or scenario geometry.

MAX_T   = 512;
DT      = 0.1;
YAW_EPS = 1e-6;

SIGMA_A = 3.0;
QPSD    = SIGMA_A*SIGMA_A;

P_FLOOR_POS = 1e-6;
P_FLOOR_VEL = 1e-7;

EGO_VAR_POS = 0.0;
EGO_VAR_YAW = 0.0;

trkState  = zeros(MAX_T, 4);
trkCov    = zeros(MAX_T, 10);
trkID     = zeros(MAX_T, 1, 'uint32');
trkStatus = zeros(MAX_T, 1, 'uint8');
nextID    = prevNextID;
if nextID < 1
    nextID = uint32(1);
end
egoTransform = zeros(1,3);
predDiag     = zeros(1,3);

speed   = egoKin(1);
yawRate = egoKin(2);
if ~isfinite(speed),   speed   = 0; end
if ~isfinite(yawRate), yawRate = 0; end

if abs(yawRate) > YAW_EPS
    dx = (speed/yawRate) * sin(yawRate*DT);
    dy = (speed/yawRate) * (1 - cos(yawRate*DT));
else
    dx = speed*DT;
    dy = 0;
end
dpsi = yawRate*DT;

egoTransform(1) = dx;
egoTransform(2) = dy;
egoTransform(3) = dpsi;

ca = cos(dpsi);
sa = sin(dpsi);
r11 =  ca;  r12 = sa;
r21 = -sa;  r22 = ca;

F = [1 0 DT 0; 0 1 0 DT; 0 0 1 0; 0 0 0 1];
Q = QPSD * [DT^4/4 0      DT^3/2 0; ...
            0      DT^4/4 0      DT^3/2; ...
            DT^3/2 0      DT^2   0; ...
            0      DT^3/2 0      DT^2];

nAct = 0; nFloor = 0; nReset = 0;

for t = 1:MAX_T
    trkID(t)     = prevID(t);
    trkStatus(t) = prevStatus(t);

    if prevStatus(t) == 0
        continue
    end
    nAct = nAct + 1;

    px = prevState(t,1) - dx;
    py = prevState(t,2) - dy;
    vx = prevState(t,3);
    vy = prevState(t,4);
    x1 = r11*px + r12*py;
    x2 = r21*px + r22*py;
    x3 = r11*vx + r12*vy;
    x4 = r21*vx + r22*vy;

    P = zeros(4,4);
    P(1,1)=prevCov(t,1); P(1,2)=prevCov(t,2); P(1,3)=prevCov(t,3); P(1,4)=prevCov(t,4);
    P(2,2)=prevCov(t,5); P(2,3)=prevCov(t,6); P(2,4)=prevCov(t,7);
    P(3,3)=prevCov(t,8); P(3,4)=prevCov(t,9);
    P(4,4)=prevCov(t,10);
    P(2,1)=P(1,2); P(3,1)=P(1,3); P(4,1)=P(1,4);
    P(3,2)=P(2,3); P(4,2)=P(2,4); P(4,3)=P(3,4);

    T = zeros(4,4);
    T(1,1)=r11; T(1,2)=r12; T(2,1)=r21; T(2,2)=r22;
    T(3,3)=r11; T(3,4)=r12; T(4,3)=r21; T(4,4)=r22;
    P = T*P*T';

    P(1,1) = P(1,1) + EGO_VAR_POS;
    P(2,2) = P(2,2) + EGO_VAR_POS;
    rr = prevState(t,1)*prevState(t,1) + prevState(t,2)*prevState(t,2);
    P(1,1) = P(1,1) + EGO_VAR_YAW*rr;
    P(2,2) = P(2,2) + EGO_VAR_YAW*rr;

    xv = [x1; x2; x3; x4];
    xv = F*xv;
    P  = F*P*F' + Q;
    P  = (P + P')/2;

    fl = false;
    if P(1,1) < P_FLOOR_POS, P(1,1) = P_FLOOR_POS; fl = true; end
    if P(2,2) < P_FLOOR_POS, P(2,2) = P_FLOOR_POS; fl = true; end
    if P(3,3) < P_FLOOR_VEL, P(3,3) = P_FLOOR_VEL; fl = true; end
    if P(4,4) < P_FLOOR_VEL, P(4,4) = P_FLOOR_VEL; fl = true; end
    if fl, nFloor = nFloor + 1; end

    okPos = isPD2(P(1,1), P(2,2), P(1,2));
    okVel = isPD2(P(3,3), P(4,4), P(3,4));
    if ~(okPos && okVel)
        d1 = P(1,1); d2 = P(2,2); d3 = P(3,3); d4 = P(4,4);
        if ~isfinite(d1) || d1 < P_FLOOR_POS, d1 = P_FLOOR_POS; end
        if ~isfinite(d2) || d2 < P_FLOOR_POS, d2 = P_FLOOR_POS; end
        if ~isfinite(d3) || d3 < P_FLOOR_VEL, d3 = P_FLOOR_VEL; end
        if ~isfinite(d4) || d4 < P_FLOOR_VEL, d4 = P_FLOOR_VEL; end
        P = zeros(4,4);
        P(1,1)=d1; P(2,2)=d2; P(3,3)=d3; P(4,4)=d4;
        nReset = nReset + 1;
    end

    trkState(t,1)=xv(1); trkState(t,2)=xv(2); trkState(t,3)=xv(3); trkState(t,4)=xv(4);
    trkCov(t,1)=P(1,1); trkCov(t,2)=P(1,2); trkCov(t,3)=P(1,3); trkCov(t,4)=P(1,4);
    trkCov(t,5)=P(2,2); trkCov(t,6)=P(2,3); trkCov(t,7)=P(2,4);
    trkCov(t,8)=P(3,3); trkCov(t,9)=P(3,4);
    trkCov(t,10)=P(4,4);
end

predDiag(1) = nAct;
predDiag(2) = nFloor;
predDiag(3) = nReset;

end

% ===========================================================================
function tf = isPD2(a, b, c)
% 2x2 symmetric [a c; c b] is positive definite iff a > 0 and det > 0.
tf = false;
if isfinite(a) && isfinite(b) && isfinite(c)
    if a > 0 && b > 0 && (a*b - c*c) > 0
        tf = true;
    end
end
end
